simulink model "PIDideal_ogr"  (Simulink 7.7)
settings: Solver=ode5  StartTime=0.0  StopTime=30  FixedStep=0.001  RelTol=1e-3
undefined symbols (not defined in the file or in its folder): Kp, Td, Ti
settings Model: Creator=koltom  LastModifiedBy=koltom  ExtModeTrigMode=oneshot  ExtModeArmWhenConnect=off
settings DataIOCC: LimitDataPoints=off
settings OptimizationCC: BlockReduction=off  BooleanDataType=off
settings DebuggingCC: SaveWithParameterizedLinksMsg=none  SignalResolutionControl=TryResolveAllWithWarning  SolverPrmCheckMsg=none  MultiTaskDSMMsg=warning  MultiTaskCondExecSysMsg=none  StrictBusMsg=None
settings HardwareCC: TargetUnknown=on
settings RTWCC: IncludeERTFirstTime=on

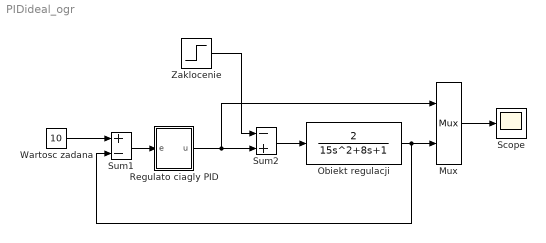
== system PIDideal_ogr ==
  Mux : Mux  Inputs=2
  Obiekt regulacji : TransferFcn  Numerator=[2]  Denominator=[15 8 1]
  Regulato ciagly PID : Subsystem
  Scope : Scope
      settings: TimeRange=30  YMin=0  YMax=16  DataFormat=Array
  Sum1 : Sum  Inputs=+-  SaturateOnIntegerOverflow=on  InputSameDT=on  OutDataTypeStr=Inherit: Same as first input
  Sum2 : Sum  Inputs=-+  SaturateOnIntegerOverflow=on  InputSameDT=on  OutDataTypeStr=Inherit: Same as first input
  Wartosc zadana : Constant  Value=10
  Zaklocenie : Step  Time=15  After=5  SampleTime=0
  wires:
  Wartosc zadana/1 -> Sum1/1
  Sum1/1 -> Regulato ciagly PID/1(e)
  Obiekt regulacji/1 -> Mux/2, Sum1/2
  Mux/1 -> Scope/1
  Regulato ciagly PID/1(u) -> Mux/1, Sum2/2
  Sum2/1 -> Obiekt regulacji/1
  Zaklocenie/1 -> Sum2/1

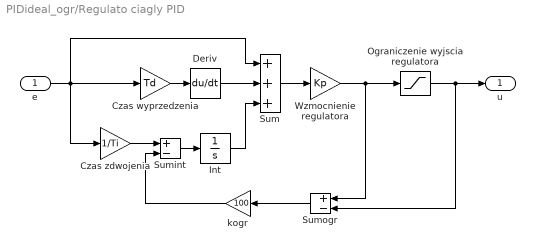
== system PIDideal_ogr/Regulato ciagly PID ==
  e : Inport
  Czas wyprzedzenia : Gain  Gain=Td  SaturateOnIntegerOverflow=on  OutDataTypeStr=Inherit: Same as input  ParamDataTypeStr=Inherit: Same as input
  Czas zdwojenia : Gain  Gain=1/Ti  SaturateOnIntegerOverflow=on  OutDataTypeStr=Inherit: Same as input  ParamDataTypeStr=Inherit: Same as input
  Deriv : Derivative
  Int : Integrator
  Ograniczenie wyjscia regulatora : Saturate  UpperLimit=15  LowerLimit=0
  Sum : Sum  Inputs=+++  SaturateOnIntegerOverflow=on  InputSameDT=on  OutDataTypeStr=Inherit: Same as first input
  Sumint : Sum  Inputs=+-  SaturateOnIntegerOverflow=on  InputSameDT=on  OutDataTypeStr=Inherit: Same as first input
  Sumogr : Sum  Inputs=+-  SaturateOnIntegerOverflow=on  InputSameDT=on  OutDataTypeStr=Inherit: Same as first input
  Wzmocnienie regulatora : Gain  Gain=Kp  SaturateOnIntegerOverflow=on  OutDataTypeStr=Inherit: Same as input  ParamDataTypeStr=Inherit: Same as input
  kogr : Gain  Gain=100  SaturateOnIntegerOverflow=on  OutDataTypeStr=Inherit: Same as input  ParamDataTypeStr=Inherit: Same as input
  u : Outport
  wires:
  e/1 -> Czas zdwojenia/1, Sum/1, Czas wyprzedzenia/1
  Sum/1 -> Wzmocnienie regulatora/1
  Wzmocnienie regulatora/1 -> Ograniczenie wyjscia regulatora/1, Sumogr/1
  Ograniczenie wyjscia regulatora/1 -> u/1, Sumogr/2
  Czas wyprzedzenia/1 -> Deriv/1
  Deriv/1 -> Sum/2
  Sumogr/1 -> kogr/1
  Sumint/1 -> Int/1
  Czas zdwojenia/1 -> Sumint/1
  kogr/1 -> Sumint/2
  Int/1 -> Sum/3
